simulink model "batteryParameterEstimation"  (R2017b)
settings: Solver=ode15s  StartTime=0  StopTime=synthData.t(end)  MaxStep=10  RelTol=1e-3  EnableMultiTasking=on
PostLoadFcn:
  | synthData_ini;
model workspace (MAT data in the model file):
  batteryParameterEstimation_spesession : sldodialogs.data.SessionData (value not decoded)
values from neighbouring files (symbols this model uses):
  SOC_LUT = (0.1:.1:1)'    [synthData_ini.m]
libraries: nesl_utility x4, fl_lib x3, pe_lib x1, simulink x1
settings Model: OrderedModelArguments=off  Creator=psanghvi  LastModifiedBy=proso
settings DataIOCC: ExternalInput=[synthData.t synthData.I]  LoadExternalInput=on  SaveFormat=Array  SignalLogging=off  DSMLogging=off
settings OptimizationCC: EnhancedBackFolding=on  ExpressionDepthLimit=2147483647  LifeSpan=1  SimCompilerOptimization=on
settings DebuggingCC: UnderspecifiedInitializationDetection=Classic  MergeDetectMultiDrivingBlocksExec=none  SolverPrmCheckMsg=warning  FcnCallInpInsideContextMsg=warning  AllowSymbolicDim=off  StateNameClashWarn=warning  SFUnexpectedBacktrackingDiag=warning  SFNoUnconditionalDefaultTransitionDiag=warning  SFExecutionAtInitializationDiag=none
settings HardwareCC: ProdBitPerPointer=32  ProdBitPerSizeT=32  ProdBitPerPtrDiffT=32  ProdLargestAtomicFloat=None  ProdIntDivRoundTo=Undefined  ProdEndianess=Unspecified  ProdWordSize=32  ProdHWDeviceType=32-bit Generic
settings ModelReferenceCC: PropagateSignalLabelsOutOfModel=off
settings SFSimCC: MATLABDynamicMemAlloc=off
settings RTWCC: SystemTargetFile=ert.tlc  GenCodeOnly=on  TemplateMakefile=ert_default_tmf  GenerateReport=on  IncludeHyperlinkInReport=on  LaunchReport=on  GenerateTraceInfo=on  GenerateTraceReport=on  GenerateTraceReportSl=on  GenerateTraceReportSf=on  GenerateTraceReportEml=on
settings CodeAppCC: IgnoreCustomStorageClasses=off  CustomSymbolStrType=$N$R$M  StateflowObjectComments=on  InternalIdentifier=Classic
settings ERTTargetCC: MultiwordLength=2048  GenerateSampleERTMain=on  ERTCustomFileTemplate=example_file_process.tlc  ConvertIfToSwitch=off  SuppressUnreachableDefaultCases=off
settings ConfigComp: CovMetricSettings=dw  CovHtmlReporting=on  CovSaveCumulativeToWorkspaceVar=on  CovSaveSingleToWorkspaceVar=on  CovExternalEMLEnable=off  CovSFcnEnable=off
settings SimscapeCC: SimscapeNormalizeSystem=off

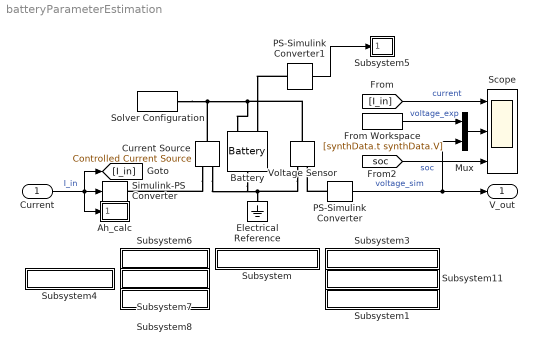
== system batteryParameterEstimation ==
  Current : Inport
  Ah_calc : Subsystem
  Battery : pe_lib/Sources/Battery  Vnom=12 V  R1=2 Ohm  prm_AH=1  AH=50 hr*A  V1=11.5 V  AH1=25 hr*A  prm_R2=1  R2=2000 Ohm  prm_fade=1  N_fade=100  AH_fade=45 hr*A  R1_fade=2.02 Ohm  V1_fade=10.35 V  i_specify=off  i_priority=None  i=0 A  i_nominal_specify=off  i_nominal_unit=A  i_nominal_value=1  v_specify=off  v_priority=None  v=0 V  v_nominal_specify=off  v_nominal_unit=V  v_nominal_value=1  charge_specify=off  charge_priority=High  charge=50 hr*A  charge_nominal_specify=off  charge_nominal_unit=hr*A  charge_nominal_value=1  num_cycles_specify=off  num_cycles_priority=High  num_cycles=0  num_cycles_nominal_specify=off  num_cycles_nominal_unit=1  num_cycles_nominal_value=1  thermal_mass=30000 J/K  Tmeas=298.15 K  Vnom_T2=12 V  R1_T2=2.2 Ohm  V1_T2=11.4 V  R2_T2=2200 Ohm  Tmeas2=273.15 K  temperature_specify=off  temperature_priority=High  temperature=298.15 K  temperature_nominal_specify=off  temperature_nominal_unit=K  temperature_nominal_value=1
      settings: SourceProductName=Simscape Power Systems  SourceProductBaseCode=PS
  Current Source : fl_lib/Electrical/Electrical Sources/Controlled Current Source
  Electrical Reference : fl_lib/Electrical/Electrical Elements/Electrical Reference
  From Workspace : FromWorkspace  VariableName=[synthData.t synthData.V]  SampleTime=0
      mask Display: disp('V_exp')
  Mux : Mux  Inputs=2
  PS-Simulink Converter : nesl_utility/PS-Simulink Converter  PhysicalDomain=network_engine_domain  SubClassName=ps_output  LeftPortType=input  RightPortType=output  PseudoPeriodic=off  Frequencies=[]  Unit=V  AffineConversion=off
  PS-Simulink Converter1 : nesl_utility/PS-Simulink Converter  PhysicalDomain=network_engine_domain  SubClassName=ps_output  LeftPortType=input  RightPortType=output  PseudoPeriodic=off  Frequencies=[]  Unit=1  AffineConversion=off
  Scope : Scope  NumInputPorts=3
  Simulink-PS Converter : nesl_utility/Simulink-PS Converter  PhysicalDomain=network_engine_domain  SubClassName=ps_input  LeftPortType=input  RightPortType=output  PseudoPeriodic=off  Frequencies=[]  NoiseDistribution=none  NoiseParameters=[]  Unit=A  AffineConversion=off  FilteringAndDerivatives=zero  SimscapeFilterOrder=1  InputFilterTimeConstant=.001  UdotUserProvided=0
  Solver Configuration : nesl_utility/Solver Configuration  PhysicalDomain=network_engine_domain  SubClassName=solver  LeftPortType=input  RightPortType=generic  Accelerate=off  Tones=[]  Harmonics=[]  SimulateNoise=off  Profile=off  UseLocalSampling=off  EnableSwitchedLinearOptims=on  FrequencyDomain=off  UseCCode=off  RelTol=0.001  AbsTol=1e-06  MinStep=1e-09  ToWorkspace=off  RevertToSquareIcSolve=off  NumHomotopyIterations=100  PhasorMode=off  PhasorModeNumHarmonics=1  DoDC=off  ResidualTolerance=1e-9  UseLocalSolver=off  LocalSolverChoice=NE_BACKWARD_EULER_ADVANCER  LocalSolverSampleTime=10  DoFixedCost=off  MaxNonlinIter=12  MaxModeIter=2  LinearAlgebra=Sparse  DelaysMemoryBudget=1024  AutomaticFiltering=on  FilteringTimeConstant=0.001
  Subsystem : Subsystem
      settings: OpenFcn=synthData_config;
      mask Display: disp('Parameter Estimation')
  Subsystem1 : Subsystem
      settings: OpenFcn=load('synthDataFinal3RC.mat')
      mask Display: disp('Final Values 3RC 20ºC')
  Subsystem11 : Subsystem
      settings: OpenFcn=load('synthDataFinal3RC.mat')
      mask Display: disp('Final Values 1RC 20ºC')
  Subsystem3 : Subsystem
      settings: OpenFcn=synthData_ini
      mask Display: disp('Initial Values')
  Subsystem4 : Subsystem
      settings: OpenFcn=|
      | figure
      | subplot(2,1,1)
      | plot(synthData.t, synthData.I)
      | ylabel('current (A)')
      | subplot(2,1,2)
      | plot(synthData.t, synthData.V)
      | ylabel('voltage (V)')
      | xlabel('time (s)')
      | p = get_param('batteryParameterEstimation','FastRestart');
      | switch p
      |     case 'on'
      |     set_param('batteryParameterEstimation','FastRestart','off')
      | end
      | % estimExp = 1;
      mask Display: disp('20ºC')
  Subsystem5 : Subsystem
  Subsystem6 : Subsystem
      settings: OpenFcn=|
      | p = get_param('batteryParameterEstimation','FastRestart');
      | switch p
      |     case 'on'
      |     set_param('batteryParameterEstimation','FastRestart','off')
      | end
      | numTau = 1;
      | synthData_config;
      mask Display: disp('1 time constant')
  Subsystem7 : Subsystem
      settings: OpenFcn=|
      | p = get_param('batteryParameterEstimation','FastRestart');
      | switch p
      |     case 'on'
      |     set_param('batteryParameterEstimation','FastRestart','off')
      | end
      | numTau = 2;
      | synthData_config;
      mask Display: disp('2 time constants')
  Subsystem8 : Subsystem
      settings: OpenFcn=|
      | p = get_param('batteryParameterEstimation','FastRestart');
      | switch p
      |     case 'on'
      |     set_param('batteryParameterEstimation','FastRestart','off')
      | end
      | numTau = 3;
      | synthData_config;
      mask Display: disp('3 time constants')
  Voltage Sensor : fl_lib/Electrical/Electrical Sensors/Voltage Sensor
  V_out : Outport
  wires:
  PS-Simulink Converter/1 -> V_out/1, Mux/2  "voltage_sim"
  Current/1 -> Ah_calc/1(I_in), [I_in], Simulink-PS Converter/1  "I_in"
  [I_in] -> Scope/1  "current"
  From Workspace/1 -> Mux/1  "voltage_exp"
  Mux/1 -> Scope/2
  [soc] -> Scope/3  "soc"
  PS-Simulink Converter1/1 -> Subsystem5/1(soc)
  connections:
  Current Source/RConn1 -- Simulink-PS Converter/RConn1
  Current Source/LConn1 -- Battery/LConn1 -- Voltage Sensor/LConn1 -- Solver Configuration/RConn1
  PS-Simulink Converter/LConn1 -- Voltage Sensor/RConn1
  Voltage Sensor/RConn2 -- Battery/RConn1 -- Current Source/RConn2 -- Electrical Reference/LConn1
  PS-Simulink Converter1/LConn1 -- Battery/LConn2

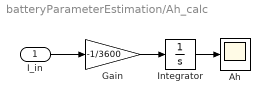
== system batteryParameterEstimation/Ah_calc ==
  I_in : Inport
  "Ah " : Scope
  Gain : Gain  Gain=-1/3600
  Integrator : Integrator
  wires:
  I_in/1 -> Gain/1
  Integrator/1 -> "Ah "/1
  Gain/1 -> Integrator/1

== system batteryParameterEstimation/Subsystem ==

== system batteryParameterEstimation/Subsystem1 ==

== system batteryParameterEstimation/Subsystem11 ==

== system batteryParameterEstimation/Subsystem3 ==

== system batteryParameterEstimation/Subsystem4 ==

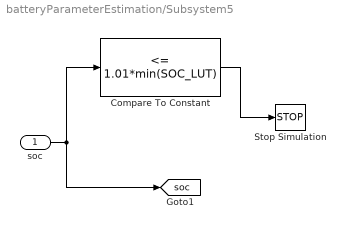
== system batteryParameterEstimation/Subsystem5 ==
  soc : Inport
  Compare To Constant : simulink/Logic and Bit Operations/Compare To Constant  relop=<=  const=1.01*min(SOC_LUT)  OutDataTypeStr=boolean
  Stop Simulation : Stop
  tag scope: soc=global
  wires:
  soc/1 -> Compare To Constant/1, [soc]
  Compare To Constant/1 -> Stop Simulation/1

== system batteryParameterEstimation/Subsystem6 ==

== system batteryParameterEstimation/Subsystem7 ==

== system batteryParameterEstimation/Subsystem8 ==
